simulink model "PX4OutputMappingC172pJSBSim"  (R2026a)
settings: configuration reference "standardSILConfiguraitonParams" (kept outside this file)
undefined symbols (not defined in the file or in its folder): ServosCommandFixedwingPlaneBus
settings Model: Creator=jerem  LastModifiedBy=Edison Altamirano
settings ConfigSetRef: SourceName=standardSILConfiguraitonParams  SourceLocation=Base Workspace

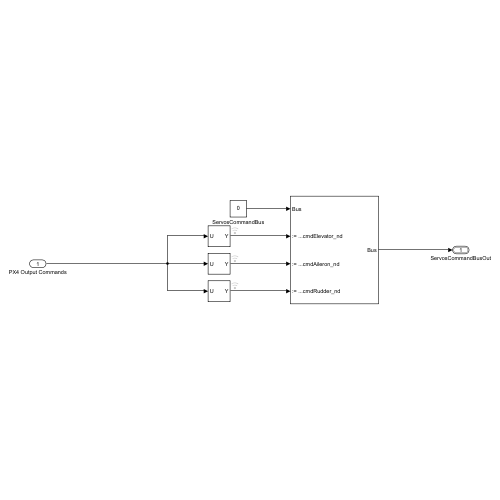
[thumbnail: Simulink's stored preview of the top-level diagram]
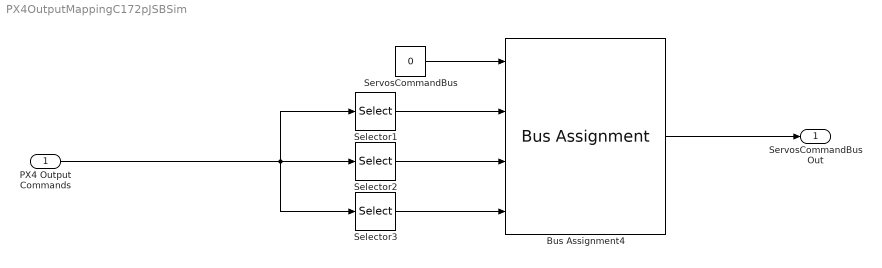
== system PX4OutputMappingC172pJSBSim ==
  PX4 Output Commands : Inport  PortDimensions=16
  Bus Assignment4 : BusAssignment  AssignedSignals=ServosCommandFixedwingPlaneBus.cmdElevator_nd,ServosCommandFixedwingPlaneBus.cmdAileron_nd,ServosCommandFixedwingPlaneBus.cmdRudder_nd
  Selector1 : Selector  InputPortWidth=16  IndexOptions=Index vector (dialog)  Indices=3  OutputSizes=1
  Selector2 : Selector  InputPortWidth=16  IndexOptions=Index vector (dialog)  Indices=2  OutputSizes=1
  Selector3 : Selector  InputPortWidth=16  IndexOptions=Index vector (dialog)  Indices=4  OutputSizes=1
  ServosCommandBus : Constant  Value=0  OutDataTypeStr=Bus: ServosCommandBus
  ServosCommandBusOut : Outport  OutDataTypeStr=Bus: ServosCommandBus
  wires:
  Selector2/1 -> Bus Assignment4/3
  Selector3/1 -> Bus Assignment4/4
  Bus Assignment4/1 -> ServosCommandBusOut/1
  Selector1/1 -> Bus Assignment4/2
  ServosCommandBus/1 -> Bus Assignment4/1
  PX4 Output Commands/1 -> Selector3/1, Selector1/1, Selector2/1
